simulink model "pole_placement_delay"  (R2017a)
settings: Solver=VariableStepAuto  StartTime=0.0  StopTime=4  RelTol=1e-3
values from neighbouring files (symbols this model uses):
  A_pp = [A5d B5d; 0 0 0 0]    [q13.m]
  B_pp = [0; 0; 0; 1]    [q13.m]
  C_pp = [C5d 0]    [q13.m]
  DCgain5 = D5d + C5cl*inv(eye(3)-A5cl)*B5d    [q13.m]    (also in q5.m; q5_reduced.m)
  DCgain_pp = D5d + C_pp_cl*inv(eye(4)-A_pp_cl)*B_pp    [q13.m]
  h5 = 2.5*pi/w    [q13.m]    (also in q5.m = 2*pi/w; q5_reduced.m = 2*pi/w)
  K5_discr = place(A5d, B5d, P_discr)    [q13.m]    (also in q5.m; q5_reduced.m)
  K_pp = place(A_pp, B_pp, P_pp_d)    [q13.m]
undefined symbols (not defined in the file or in its folder): A5d, B5d, C5d, D5d
settings Model: Creator=Aleksandra  LastModifiedBy=Aleksandra

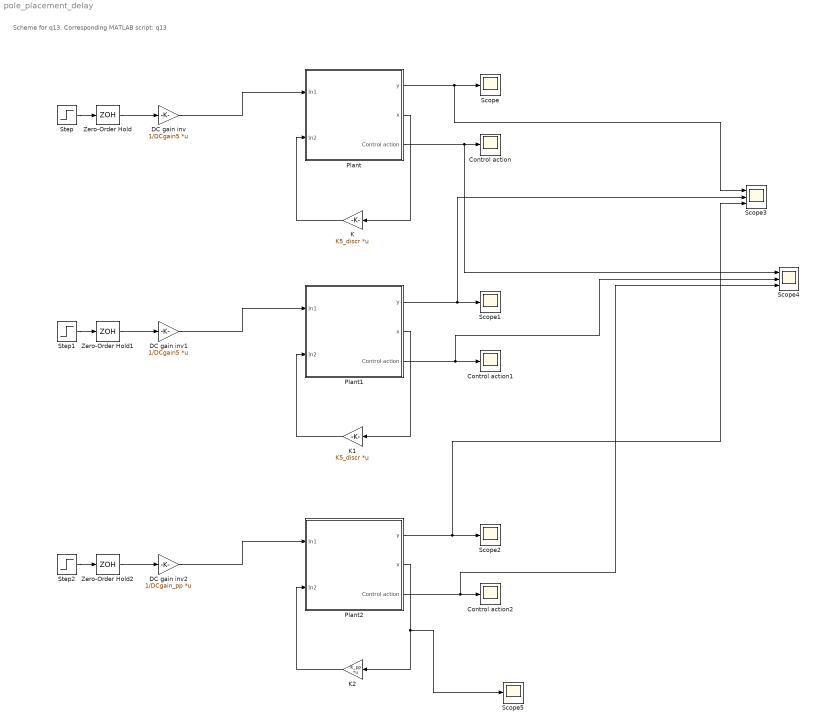
== system pole_placement_delay ==
  note: Scheme for q13.
      | Corresponding MATLAB script: q13
  Control action : Scope
  Control action1 : Scope
  Control action2 : Scope
  DC gain inv : Gain  Gain=1/DCgain5  Multiplication=Matrix(K*u)
  DC gain inv1 : Gain  Gain=1/DCgain5  Multiplication=Matrix(K*u)
  DC gain inv2 : Gain  Gain=1/DCgain_pp  Multiplication=Matrix(K*u)
  K : Gain  Gain=K5_discr  Multiplication=Matrix(K*u)
  K1 : Gain  Gain=K5_discr  Multiplication=Matrix(K*u)
  K2 : Gain  Gain=K_pp  Multiplication=Matrix(K*u)
  Plant : Subsystem
  Plant1 : Subsystem
  Plant2 : Subsystem
  Scope{,1..2,5} (4 alike) : Scope
  Scope3 : Scope  NumInputPorts=3
  Scope4 : Scope  NumInputPorts=3
  Step : Step  Time=0  SampleTime=0
  Step1 : Step  Time=0  SampleTime=0
  Step2 : Step  Time=0  SampleTime=0
  Zero-Order Hold : ZeroOrderHold  SampleTime=h5
  Zero-Order Hold1 : ZeroOrderHold  SampleTime=h5
  Zero-Order Hold2 : ZeroOrderHold  SampleTime=h5
  wires:
  Step/1 -> Zero-Order Hold/1
  DC gain inv/1 -> Plant/1(In1)
  Plant/1(y) -> Scope3/1, Scope/1
  Plant/2(x) -> K/1
  K/1 -> Plant/2(In2)
  Zero-Order Hold/1 -> DC gain inv/1
  Plant/3(Control action) -> Scope4/1, Control action/1
  Plant1/1(y) -> Scope3/2, Scope1/1
  Zero-Order Hold1/1 -> DC gain inv1/1
  Step1/1 -> Zero-Order Hold1/1
  Plant1/2(x) -> K1/1
  Plant1/3(Control action) -> Scope4/2, Control action1/1
  K1/1 -> Plant1/2(In2)
  DC gain inv1/1 -> Plant1/1(In1)
  K2/1 -> Plant2/2(In2)
  Plant2/2(x) -> Scope5/1, K2/1
  Plant2/3(Control action) -> Scope4/3, Control action2/1
  DC gain inv2/1 -> Plant2/1(In1)
  Zero-Order Hold2/1 -> DC gain inv2/1
  Step2/1 -> Zero-Order Hold2/1
  Plant2/1(y) -> Scope3/3, Scope2/1

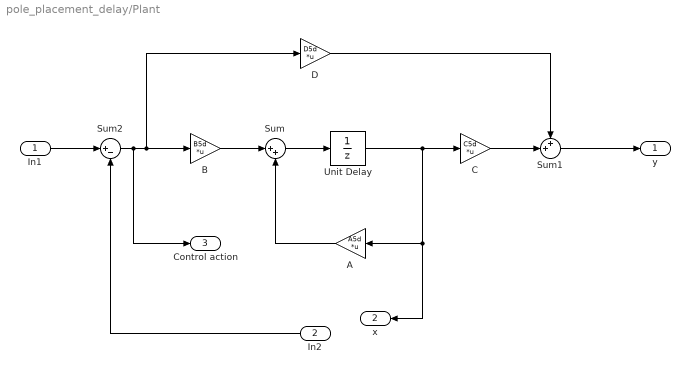
== system pole_placement_delay/Plant ==
  In1 : Inport
  In2 : Inport  Port=2
  A : Gain  Gain=A5d  Multiplication=Matrix(K*u)
  B : Gain  Gain=B5d  Multiplication=Matrix(K*u)
  C : Gain  Gain=C5d  Multiplication=Matrix(K*u)
  D : Gain  Gain=D5d  Multiplication=Matrix(K*u)
  Sum : Sum  Inputs=|++
  Sum1 : Sum  Inputs=++|
  Sum2 : Sum  Inputs=|+-
  Unit Delay : UnitDelay  SampleTime=-1
  y : Outport
  x : Outport  Port=2
  Control action : Outport  Port=3
  wires:
  Sum/1 -> Unit Delay/1
  A/1 -> Sum/2
  D/1 -> Sum1/1
  C/1 -> Sum1/2
  Sum1/1 -> y/1
  B/1 -> Sum/1
  Sum2/1 -> Control action/1, D/1, B/1
  Unit Delay/1 -> x/1, A/1, C/1
  In2/1 -> Sum2/2
  In1/1 -> Sum2/1

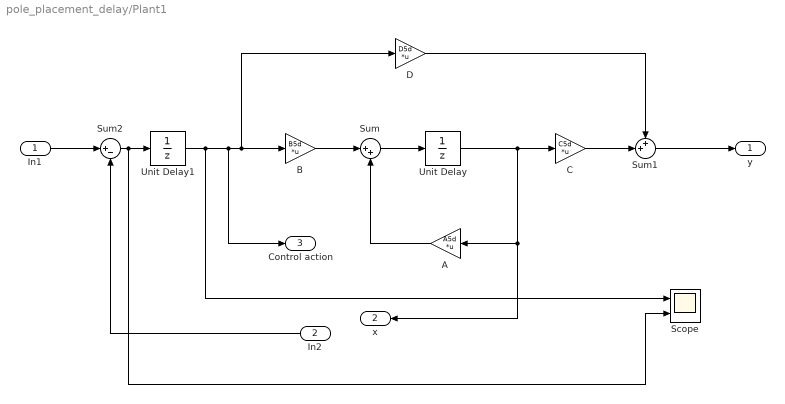
== system pole_placement_delay/Plant1 ==
  In1 : Inport
  In2 : Inport  Port=2
  A : Gain  Gain=A5d  Multiplication=Matrix(K*u)
  B : Gain  Gain=B5d  Multiplication=Matrix(K*u)
  C : Gain  Gain=C5d  Multiplication=Matrix(K*u)
  D : Gain  Gain=D5d  Multiplication=Matrix(K*u)
  Scope : Scope  NumInputPorts=2
  Sum : Sum  Inputs=|++
  Sum1 : Sum  Inputs=++|
  Sum2 : Sum  Inputs=|+-
  Unit Delay : UnitDelay  SampleTime=-1
  Unit Delay1 : UnitDelay  SampleTime=h5
  y : Outport
  x : Outport  Port=2
  Control action : Outport  Port=3
  wires:
  Sum/1 -> Unit Delay/1
  A/1 -> Sum/2
  D/1 -> Sum1/1
  C/1 -> Sum1/2
  Sum1/1 -> y/1
  B/1 -> Sum/1
  Sum2/1 -> Scope/2, Unit Delay1/1
  Unit Delay/1 -> x/1, A/1, C/1
  In2/1 -> Sum2/2
  In1/1 -> Sum2/1
  Unit Delay1/1 -> Scope/1, Control action/1, D/1, B/1

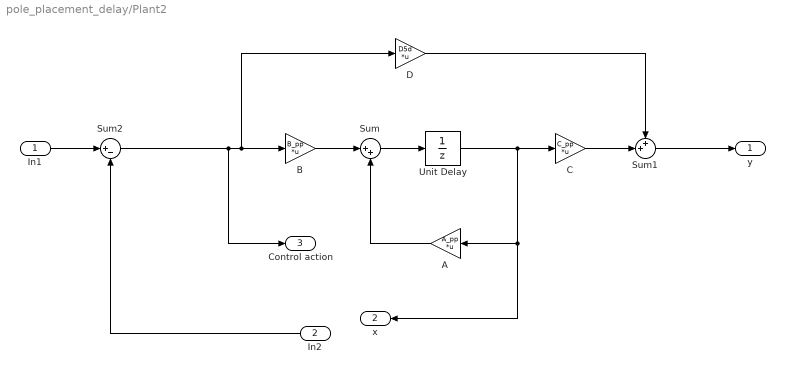
== system pole_placement_delay/Plant2 ==
  In1 : Inport
  In2 : Inport  Port=2
  A : Gain  Gain=A_pp  Multiplication=Matrix(K*u)
  B : Gain  Gain=B_pp  Multiplication=Matrix(K*u)
  C : Gain  Gain=C_pp  Multiplication=Matrix(K*u)
  D : Gain  Gain=D5d  Multiplication=Matrix(K*u)
  Sum : Sum  Inputs=|++
  Sum1 : Sum  Inputs=++|
  Sum2 : Sum  Inputs=|+-
  Unit Delay : UnitDelay  SampleTime=-1
  y : Outport
  x : Outport  Port=2
  Control action : Outport  Port=3
  wires:
  Sum/1 -> Unit Delay/1
  A/1 -> Sum/2
  D/1 -> Sum1/1
  C/1 -> Sum1/2
  Sum1/1 -> y/1
  B/1 -> Sum/1
  Unit Delay/1 -> x/1, A/1, C/1
  In2/1 -> Sum2/2
  In1/1 -> Sum2/1
  Sum2/1 -> Control action/1, D/1, B/1
